simulink model "step1"  (R2021a)
settings: Solver=FixedStepAuto  StartTime=0.0  StopTime=10.0  FixedStep=0.001  RelTol=1e-3
settings Model: Creator=konsta  LastModifiedBy=konsta

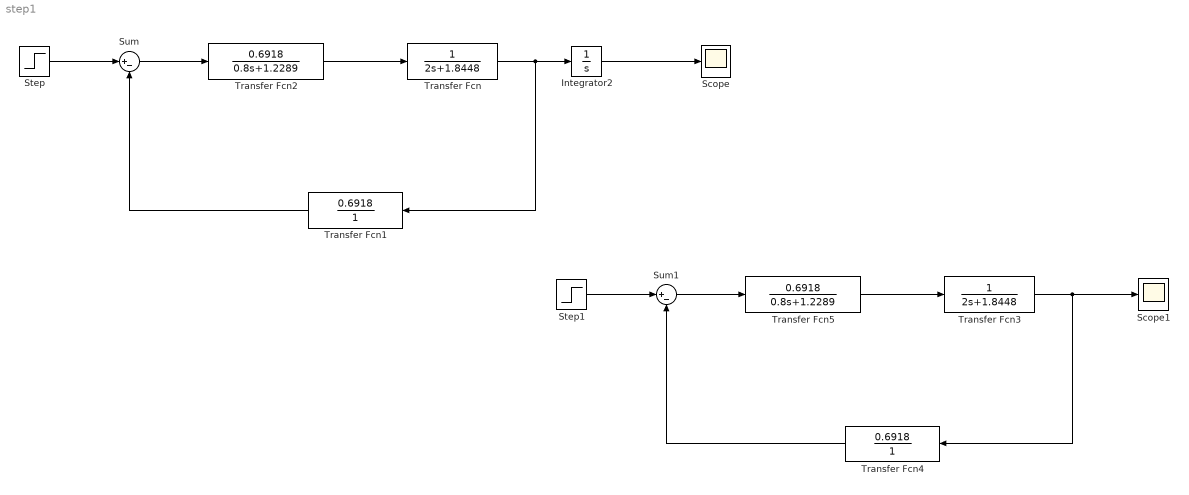
== system step1 ==
  Integrator2 : Integrator
  Scope : Scope
  Scope1 : Scope
  Step : Step  SampleTime=0
  Step1 : Step  SampleTime=0
  Sum : Sum  Inputs=|+-
  Sum1 : Sum  Inputs=|+-
  Transfer Fcn : TransferFcn  Denominator=[2 1.8448]
  Transfer Fcn1 : TransferFcn  Numerator=[0.6918]  Denominator=[0 1]
  Transfer Fcn2 : TransferFcn  Numerator=[0.6918]  Denominator=[0.8 1.2289]
  Transfer Fcn3 : TransferFcn  Denominator=[2 1.8448]
  Transfer Fcn4 : TransferFcn  Numerator=[0.6918]  Denominator=[0 1]
  Transfer Fcn5 : TransferFcn  Numerator=[0.6918]  Denominator=[0.8 1.2289]
  wires:
  Step/1 -> Sum/1
  Integrator2/1 -> Scope/1
  Sum/1 -> Transfer Fcn2/1
  Transfer Fcn2/1 -> Transfer Fcn/1
  Transfer Fcn/1 -> Transfer Fcn1/1, Integrator2/1
  Transfer Fcn1/1 -> Sum/2
  Sum1/1 -> Transfer Fcn5/1
  Transfer Fcn4/1 -> Sum1/2
  Transfer Fcn3/1 -> Scope1/1, Transfer Fcn4/1
  Step1/1 -> Sum1/1
  Transfer Fcn5/1 -> Transfer Fcn3/1
